simulink model "linear_yaw_control_R2015a_part_b"  (R2015b)
settings: Solver=ode45  StartTime=0.0  StopTime=10.0  RelTol=1e-3
values from neighbouring files (symbols this model uses):
  a = 50    [RunSimLab7[Conflict].m]
  kpr = [-7]    [RunSimLab7.m]    (also in RunSimLab7[Conflict].m)
  numP_r_from_dr = numPdr(3,:)    [RunSimLab7.m]    (also in RunSimLab7[Conflict].m)
  yaw_com = 0.5*pi/180    (= 0.00872664625997)    [RunSimLab7.m]    (also in RunSimLab7[Conflict].m = 0.0872664625997)
undefined symbols (not defined in the file or in its folder): denPdr
libraries: dspsrcs4 x1
settings Model: Creator=Eric  LastModifiedBy=Jeremy
settings DataIOCC: SaveFormat=Array
settings OptimizationCC: ExpressionDepthLimit=2147483647
settings DebuggingCC: UnderspecifiedInitializationDetection=Classic  MergeDetectMultiDrivingBlocksExec=none  SolverPrmCheckMsg=warning  StateNameClashWarn=warning
settings HardwareCC: ProdBitPerPointer=32  ProdLargestAtomicFloat=None  ProdIntDivRoundTo=Undefined  ProdEndianess=Unspecified  ProdWordSize=32  ProdHWDeviceType=32-bit Generic
settings GRTTargetCC: GeneratePreprocessorConditionals=Disable all
settings ConfigComp: CovModelRefEnable=Off  CovSFcnEnable=off

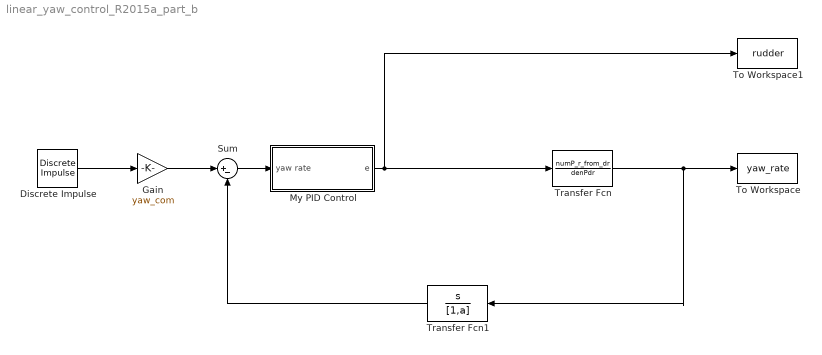
== system linear_yaw_control_R2015a_part_b ==
  Discrete Impulse : dspsrcs4/Discrete  Impulse  Delay=1  SampleTime=1  FrameSample=1  OutputFrames=off  dataType=double  isSigned=on  wordLen=16  udDataType=sfix(16)  fracBitsMode=Best precision  numFracBits=15  OutDataTypeStr=double  LastOutDataTypeStr=double
  Gain : Gain  Gain=yaw_com
  My PID Control : Subsystem  TreatAsAtomicUnit=on
  Sum : Sum  Inputs=|+-
  To Workspace : ToWorkspace  VariableName=yaw_rate  SaveFormat=Timeseries  SampleTime=-1
  To Workspace1 : ToWorkspace  VariableName=rudder  SaveFormat=Timeseries  SampleTime=-1
  Transfer Fcn : TransferFcn  Numerator=numP_r_from_dr  Denominator=denPdr
  Transfer Fcn1 : TransferFcn  Numerator=[1,0]  Denominator=[1,a]
  wires:
  Transfer Fcn/1 -> Transfer Fcn1/1, To Workspace/1
  Discrete Impulse/1 -> Gain/1
  Gain/1 -> Sum/1
  Sum/1 -> My PID Control/1(yaw rate)
  My PID Control/1(e) -> To Workspace1/1, Transfer Fcn/1
  Transfer Fcn1/1 -> Sum/2

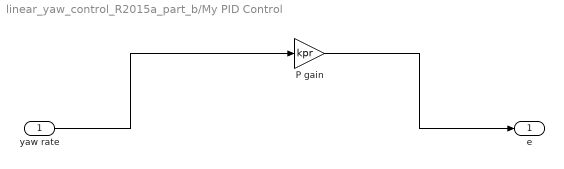
== system linear_yaw_control_R2015a_part_b/My PID Control ==
  yaw rate : Inport
  P gain : Gain  Gain=kpr
  e : Outport
  wires:
  yaw rate/1 -> P gain/1
  P gain/1 -> e/1
